simulink model "SerializerTest"  (R2015b)
settings: Solver=VariableStepAuto  StartTime=0.0  StopTime=10.0  RelTol=1e-3
libraries: commrandsrc3 x3, simulink x1, aerolibanimutils x1
settings Model: Creator=Ryuu  LastModifiedBy=Ryuu

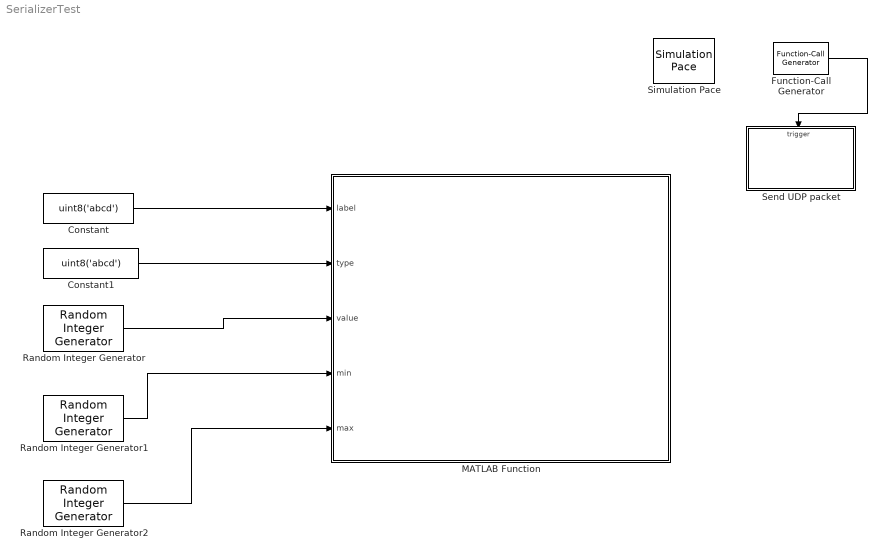
== system SerializerTest ==
  Constant : Constant  Value=uint8('abcd')
  Constant1 : Constant  Value=uint8('abcd')
  Function-Call Generator : simulink/Ports & Subsystems/Function-Call Generator  sample_time=.5  numberOfIterations=1
  MATLAB Function : MATLAB Function  TreatAsAtomicUnit=on
  Random Integer Generator : commrandsrc3/Random Integer Generator  SetSize=1000  SeedSource=Auto  Seed=0  SampleTime=0.01  SamplesPerFrame=200  OutputDataType=double  SimulateUsing=Interpreted execution
  Random Integer Generator1 : commrandsrc3/Random Integer Generator  SetSize=1000  SeedSource=Auto  Seed=0  SampleTime=0.01  SamplesPerFrame=200  OutputDataType=double  SimulateUsing=Interpreted execution
  Random Integer Generator2 : commrandsrc3/Random Integer Generator  SetSize=1000  SeedSource=Auto  Seed=0  SampleTime=0.01  SamplesPerFrame=200  OutputDataType=double  SimulateUsing=Interpreted execution
  Send UDP packet : Subsystem
  Simulation Pace : aerolibanimutils/Simulation Pace  SimulationPace=1  SleepMode=MATLAB Thread  OutputPaceError=off  SampleTime=1/30
  wires:
  Function-Call Generator/1 -> Send UDP packet/Trigger
  Random Integer Generator/1 -> MATLAB Function/3(value)
  Random Integer Generator1/1 -> MATLAB Function/4(min)
  Random Integer Generator2/1 -> MATLAB Function/5(max)
  Constant/1 -> MATLAB Function/1(label)
  Constant1/1 -> MATLAB Function/2(type)

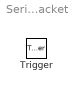
== system SerializerTest/Send UDP packet ==
  Trigger : TriggerPort  TriggerType=function-call  PortDimensions=1

== matlab function SerializerTest/MATLAB Function ==
  data: label input; type input; value input; min input; max input
function data_serialize(label, type, value, min, max)

label_ser = sensor_serialize(label);
type_ser = sensor_serialize(type);
value_ser = sensor_serialize(value);
min_ser = sensor_serialize(min);
max_ser = sensor_serialize(max);


V = length(label_ser);
W = length(type_ser);
X = length(value_ser);
Y = length(min_ser);
Z = length(max_ser);

output = [
    V;label_ser;
    W;type_ser;
    X;value_ser;
    Y;min_ser;
    Z;max_ser;
    ];
end


function m = sensor_serialize(v)
    % dispatch according to type
    if isnumeric(v) 
        m = serialize_numeric(v);
    elseif ischar(v)
        m = serialize_string(v);
    elseif islogical(v)
        m = serialize_logical(v);
    elseif isobject(v)
        m = serialize_object(v);
    end
end

% single scalar
function m = serialize_scalar(v)
    % Data type & data
    m = [class2tag(class(v)); typecast(v,'uint8').'];
end

% char arrays
function m = serialize_string(v)
    if size(v,1) == 1
        % horizontal string: Type, Length, and Data
        m = [uint8(0); typecast(uint32(length(v)),'uint8').'; uint8(v(:))];
    elseif sum(size(v)) == 0
        % '': special encoding
        m = uint8(200);
    else
        % general char array: Tag & Number of dimensions, Dimensions, Data
        m = [uint8(132); ndims(v); typecast(uint32(size(v)),'uint8').'; uint8(v(:))];
    end
end

% logical arrays
function m = serialize_logical(v)
    % Tag & Number of dimensions, Dimensions, Data
    m = [uint8(133); ndims(v); typecast(uint32(size(v)),'uint8').'; uint8(v(:))];
end

% non-complex and non-sparse numerical matrix
function m = serialize_numeric_simple(v)
    % Tag & Number of dimensions, Dimensions, Data
    m = [16+class2tag(class(v)); ndims(v); typecast(uint32(size(v)),'uint8').'; typecast(v(:).','uint8').'];
end

% Numeric Matrix: can be real/complex, sparse/full, scalar
function m = serialize_numeric(v)
    if issparse(v)
        % Data Type & Dimensions
        m = [uint8(130); typecast(uint64(size(v,1)), 'uint8').'; typecast(uint64(size(v,2)), 'uint8').']; % vectorize
        % Index vectors
        [i,j,s] = find(v);        
        % Real/Complex
        if isreal(v)
            m = [m; serialize_numeric_simple(i); serialize_numeric_simple(j); 1; serialize_numeric_simple(s)];
        else
            m = [m; serialize_numeric_simple(i); serialize_numeric_simple(j); 0; serialize_numeric_simple(real(s)); serialize_numeric_simple(imag(s))];
        end
    elseif ~isreal(v)
        % Data type & contents
        m = [uint8(131); serialize_numeric_simple(real(v)); serialize_numeric_simple(imag(v))];
    elseif isscalar(v)
        % Scalar
        m = serialize_scalar(v);
    else
        % Simple matrix
        m = serialize_numeric_simple(v);
    end
end

% *container* class to byte
function b = class2tag(cls)
	switch cls
		case 'string'
            b = uint8(0);
		case 'double'
			b = uint8(1);
		case 'single'
			b = uint8(2);
		case 'int8'
			b = uint8(3);
		case 'uint8'
			b = uint8(4);
		case 'int16'
			b = uint8(5);
		case 'uint16'
			b = uint8(6);
		case 'int32'
			b = uint8(7);
		case 'uint32'
			b = uint8(8);
		case 'int64'
			b = uint8(9);
		case 'uint64'
			b = uint8(10);
		otherwise
			error('Unknown class');
    end
end

% emit a specific warning only once (per MATLAB session)
function warn_once(varargin)
persistent displayed_warnings;
% determine the message content
if length(varargin) > 1 && any(varargin{1}==':') && ~any(varargin{1}==' ') && ischar(varargin{2})
    message_content = [varargin{1} sprintf(varargin{2:end})];
else
    message_content = sprintf(varargin{1:end});
end
% generate a hash of of the message content
str = java.lang.String(message_content);
message_id = sprintf('x%.0f',str.hashCode()+2^31);
% and check if it had been displayed before
if ~isfield(displayed_warnings,message_id)
    % emit the warning
    warning(varargin{:});
    % remember to not display the warning again
    displayed_warnings.(message_id) = true;
end
end
